simulink model "testI2tInputData"  (R2016b)
settings: Solver=FixedStepAuto  StartTime=0.0  StopTime=180  FixedStep=0.002  RelTol=1e-3
libraries: I2tChecker x1
settings Model: DataDictionary=ModelDictionary.sldd  Creator=Marc  LastModifiedBy=Marc
settings DataIOCC: ExternalInput=ds  LoadExternalInput=on

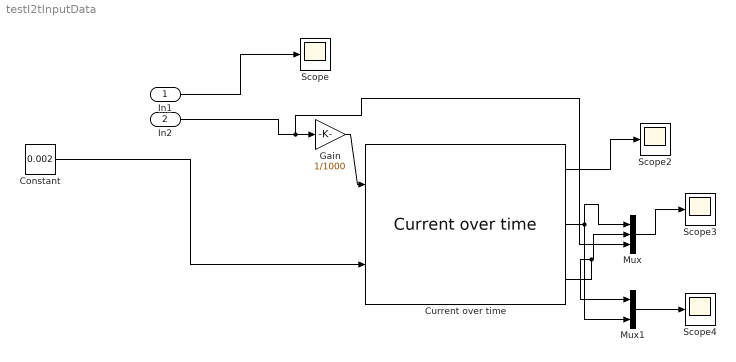
== system testI2tInputData ==
  In1 : Inport
  In2 : Inport  Port=2
  Constant : Constant  Value=0.002
  Current over time : I2tChecker/Current over time
  Gain : Gain  Gain=1/1000
  Mux : Mux  Inputs=3
  Mux1 : Mux  Inputs=2
  Scope{,2..4} (4 alike) : Scope
  wires:
  Current over time/1 -> Scope2/1
  In1/1 -> Scope/1
  In2/1 -> Mux/3, Gain/1
  Current over time/3 -> Mux1/1, Mux/2
  Mux/1 -> Scope3/1
  Current over time/2 -> Mux/1, Mux1/2
  Gain/1 -> Current over time/1
  Mux1/1 -> Scope4/1
  Constant/1 -> Current over time/2
